simulink model "lab_1_position_sim (2)"  (R2016a)
settings: Solver=VariableStepAuto  SolverMode=SingleTasking  StartTime=0.0  StopTime=10.0  RelTol=1e-3
undefined symbols (not defined in the file or in its folder): DiscIntNeverNeededParam, K, tau
libraries: simulink x2
settings Model: Creator=MSI  LastModifiedBy=MSI
settings DebuggingCC: SFUnexpectedBacktrackingDiag=error  SFNoUnconditionalDefaultTransitionDiag=error
settings SFSimCC: SimUseLocalCustomCode=on
settings RTWCC: RTWUseLocalCustomCode=on
settings GRTTargetCC: TargetLangStandard=C99 (ISO)  GeneratePreprocessorConditionals=Use local settings
settings ConfigComp: CovMetricSettings=dwe  CovHtmlReporting=off  CovSaveCumulativeToWorkspaceVar=off  CovSaveSingleToWorkspaceVar=off  CovExternalEMLEnable=on

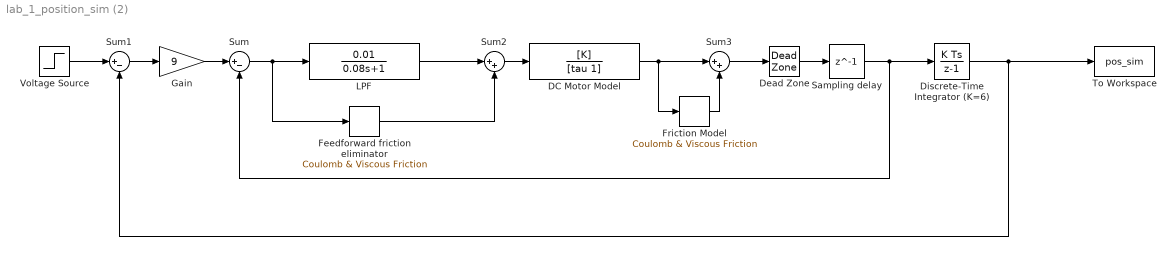
== system lab_1_position_sim (2) ==
  DC Motor Model : TransferFcn  Numerator=[K]  Denominator=[tau 1]
  Dead Zone : DeadZone  LowerValue=-10  UpperValue=10  SaturateOnIntegerOverflow=on
  Discrete-Time Integrator (K=6) : DiscreteIntegrator  gainval=6  InitialConditionSetting=State (most efficient)  SampleTime=-1  ICPrevOutput=DiscIntNeverNeededParam  ICPrevScaledInput=DiscIntNeverNeededParam
  Feedforward friction eliminator : simulink/Discontinuities/Coulomb & Viscous Friction  offset=2  gain=0
  Friction Model : simulink/Discontinuities/Coulomb & Viscous Friction  offset=-15  gain=-0.1
  Gain : Gain  Gain=9
  LPF : TransferFcn  Numerator=0.01  Denominator=[0.08 1]
  Sampling delay : Delay  DelayLength=1
  Sum : Sum  Inputs=|+-
  Sum1 : Sum  Inputs=|+-
  Sum2 : Sum  Inputs=|++
  Sum3 : Sum  Inputs=|++
  To Workspace : ToWorkspace  VariableName=pos_sim  SaveFormat=Timeseries  SampleTime=-1
  Voltage Source : Step  Time=0  After=90  SampleTime=0
  wires:
  Sum3/1 -> Dead Zone/1
  LPF/1 -> Sum2/1
  Sum1/1 -> Gain/1
  Sum2/1 -> DC Motor Model/1
  Discrete-Time Integrator (K=6)/1 -> To Workspace/1, Sum1/2
  Sum/1 -> Feedforward friction eliminator/1, LPF/1
  DC Motor Model/1 -> Friction Model/1, Sum3/1
  Friction Model/1 -> Sum3/2
  Feedforward friction eliminator/1 -> Sum2/2
  Gain/1 -> Sum/1
  Voltage Source/1 -> Sum1/1
  Dead Zone/1 -> Sampling delay/1
  Sampling delay/1 -> Discrete-Time Integrator (K=6)/1, Sum/2
